simulink subsystem "system_inputs"  (R2022b)
settings: Solver=VariableStepAuto  StartTime=0.0  StopTime=10.0  RelTol=1e-3
undefined symbols (not defined in the file): R
libraries: mbedblockslib x1
settings Model: Creator=micha  LastModifiedBy=micha
settings ModelReferenceCC: EnableRefExpFcnMdlSchedulingChecks=on

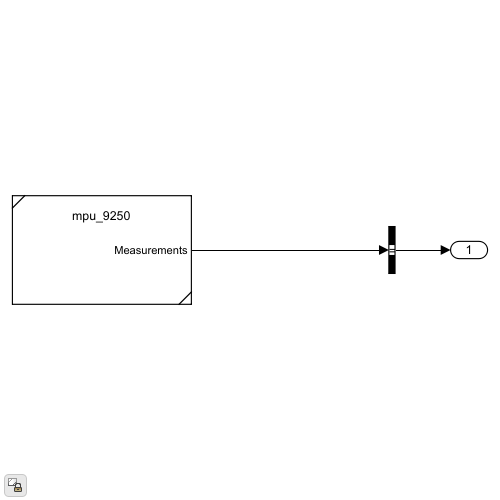
[thumbnail: Simulink's stored preview of the top-level diagram]
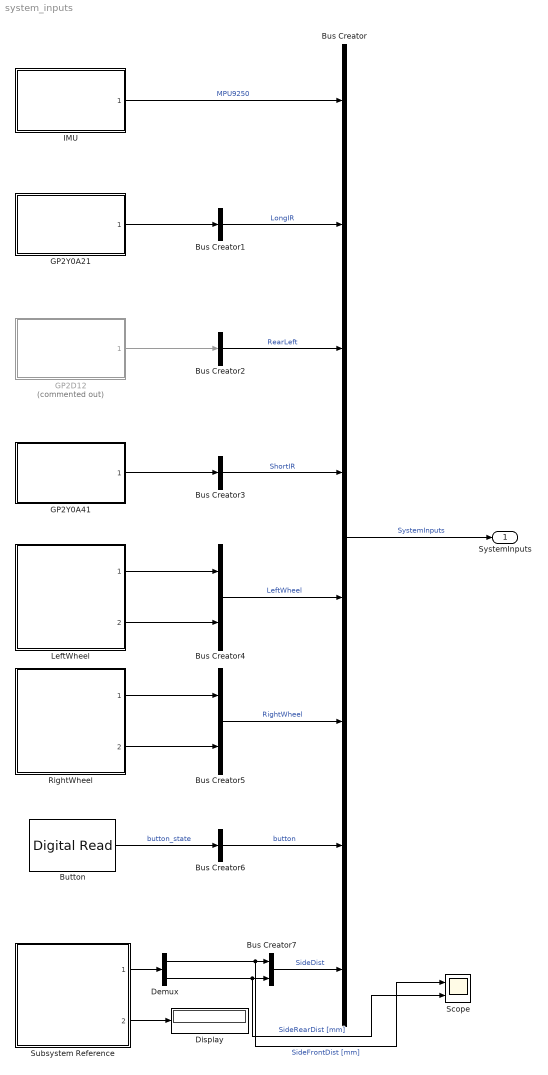
== system system_inputs ==
  Bus Creator : BusCreator  Inputs=8
  Bus Creator{1..3,6} (4 alike) : BusCreator  Inputs=1
  Bus Creator4 : BusCreator  Inputs=2
  Bus Creator5 : BusCreator  Inputs=2
  Bus Creator7 : BusCreator  Inputs=2
  Button : mbedblockslib/Digital Read  Pin=PC_13  Direction=input  SampleTime=-1
      settings: LibrarySourceBlock=stmnucleorootlib/Common/Digital Read
  Demux : Demux  Outputs=2
  Display : Display
  GP2D12 : Subsystem  Commented=on  ReferencedSubsystem=distance_sensor  Pin=PC_4  Breakpoints=[0.0290, 0.0390, 0.0600, 0.0820, 0.1340, 0.1600, 0.1810, 0.2070, 0.2330, 0.2650, 0.3030, 0.3590, 0.4460, 0.5810, 0.6870, 0.7940]  Table=[900, 800, 750, 700, 600, 550, 500, 450, 400, 350, 300, 250, 200, 150, 125, 100]
  GP2Y0A21 : Subsystem  ReferencedSubsystem=distance_sensor  Pin=PC_3  Breakpoints=[0.0830, 0.1090, 0.1230, 0.1340, 0.1560, 0.1680, 0.1820, 0.1990, 0.2210, 0.2480, 0.2860, 0.3430, 0.4260, 0.5650, 0.6730, 0.8390, 0.9460]  Table=[900, 800, 750, 700, 600, 550, 500, 450, 400, 350, 300, 250, 200, 150, 125, 100, 70]
  GP2Y0A41 : Subsystem  ReferencedSubsystem=distance_sensor  Pin=PC_2  Breakpoints=[0.0170, 0.0250, 0.0360, 0.0560, 0.0790, 0.1070, 0.1250, 0.1550, 0.2010, 0.2780, 0.3330, 0.4370, 0.6420, 0.8780]  Table=[600, 550, 500, 450, 400, 350, 300, 250, 200, 150, 125, 100, 70, 50]
  IMU : Subsystem  ReferencedSubsystem=MPU_9250
  LeftWheel : Subsystem  ReferencedSubsystem=wheel_encoder  R=R  n=24  invert=off  PinA=PB_1  PinB=PB_15
  RightWheel : Subsystem  ReferencedSubsystem=wheel_encoder  R=R  n=24  invert=on  PinA=PB_14  PinB=PB_13
  Scope : Scope  NumInputPorts=2
  Subsystem Reference : Subsystem  ReferencedSubsystem=tof_sensors  Pin=D5
  SystemInputs : Outport
  wires:
  Bus Creator/1 -> SystemInputs/1  "SystemInputs"
  IMU/1 -> Bus Creator/1  "MPU9250"
  Bus Creator1/1 -> Bus Creator/2  "LongIR"
  Bus Creator2/1 -> Bus Creator/3  "RearLeft"
  Bus Creator3/1 -> Bus Creator/4  "ShortIR"
  GP2Y0A21/1 -> Bus Creator1/1
  GP2Y0A41/1 -> Bus Creator3/1
  LeftWheel/2 -> Bus Creator4/2
  Bus Creator4/1 -> Bus Creator/5  "LeftWheel"
  Bus Creator5/1 -> Bus Creator/6  "RightWheel"
  LeftWheel/1 -> Bus Creator4/1
  RightWheel/1 -> Bus Creator5/1
  RightWheel/2 -> Bus Creator5/2
  Button/1 -> Bus Creator6/1  "button_state"
  Bus Creator6/1 -> Bus Creator/7  "button"
  GP2D12/1 -> Bus Creator2/1
  Subsystem Reference/1 -> Demux/1
  Demux/1 -> Bus Creator7/1, Scope/1  "SideFrontDist [mm]"
  Demux/2 -> Bus Creator7/2, Scope/2  "SideRearDist [mm]"
  Subsystem Reference/2 -> Display/1
  Bus Creator7/1 -> Bus Creator/8  "SideDist"
